simulink model "ESPSIM_Transmission_Multiplex"  (R2025a)
settings: Solver=ode3  StartTime=0.0  StopTime=inf  RelTol=1e-3  EnableMultiTasking=on
libraries: arduinolib x4
settings Model: FPTRunName=Active  SILPILModeSetting=veronly  ExtModeTrigDuration=2  Creator=antho  LastModifiedBy=antho
settings SolverCC: AlgebraicLoopSolver=TrustRegion  AutoInsertRateTranBlk=on
settings DataIOCC: LimitDataPoints=on  SaveFormat=Array
settings OptimizationCC: ReuseModelBlockBuffer=off  ExpressionDepthLimit=2147483647.0  LifeSpan=Inf  MaxStackSize=64
settings DebuggingCC: UnderspecifiedInitializationDetection=Classic  MergeDetectMultiDrivingBlocksExec=none  FcnCallInpInsideContextMsg=warning  UnconnectedInputMsg=warning  UnconnectedOutputMsg=warning  UnconnectedLineMsg=warning  AllowSymbolicDim=off  StateNameClashWarn=warning  SFUnexpectedBacktrackingDiag=warning  SFNoUnconditionalDefaultTransitionDiag=warning  SFExecutionAtInitializationDiag=none  ArithmeticOperatorsInVariantConditions=warning
settings HardwareCC: ProdBitPerPointer=32.0  ProdBitPerSizeT=32.0  ProdBitPerPtrDiffT=32.0  ProdLargestAtomicInteger=Long  ProdLargestAtomicFloat=Double  ProdWordSize=32.0  ProdHWDeviceType=ARM Compatible->ARM Cortex
settings ModelReferenceCC: EnableRefExpFcnMdlSchedulingChecks=on  PropagateSignalLabelsOutOfModel=off
settings SFSimCC: SimUseLocalCustomCode=off  CustomCodeUndefinedFunction=UseInterfaceOnly
settings RTWCC: SystemTargetFile=ert.tlc  HardwareBoard=ESP32-WROOM (Arduino Compatible)  TemplateMakefile=ert_default_tmf  GenerateReport=on  RTWVerbose=off  RTWUseLocalCustomCode=off  Toolchain=ESP32  BuildConfiguration=Faster Runs  LaunchReport=on  GPUComputeCapability=3.5  Description=Embedded Coder
settings CodeAppCC: ForceParamTrailComments=on  OperatorAnnotations=on  StateflowObjectComments=on  MATLABSourceComments=on
settings ERTTargetCC: ExtModeTransport=3.0  ExtModeAutomaticAllocSize=off  ExtModeStaticAllocSize=65536.0  InlinedParameterPlacement=Hierarchical  DynamicArrayContainerType=coder::array  MultiwordLength=2048.0  ERTCustomFileBanners=off  SupportContinuousTime=on  SupportNonInlinedSFcns=on  RemoveResetFunc=off  SupportVariableSizeSignals=on  ModelStepFunctionPrototypeControlCompliant=off
settings ConfigComp: CovMetricSettings=dw  CovSaveCumulativeToWorkspaceVar=on  CovSaveSingleToWorkspaceVar=on  CovExternalEMLEnable=off  CovSFcnEnable=off

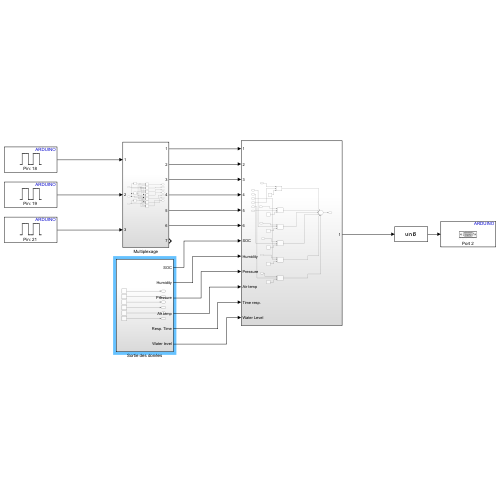
[thumbnail: Simulink's stored preview of the top-level diagram]
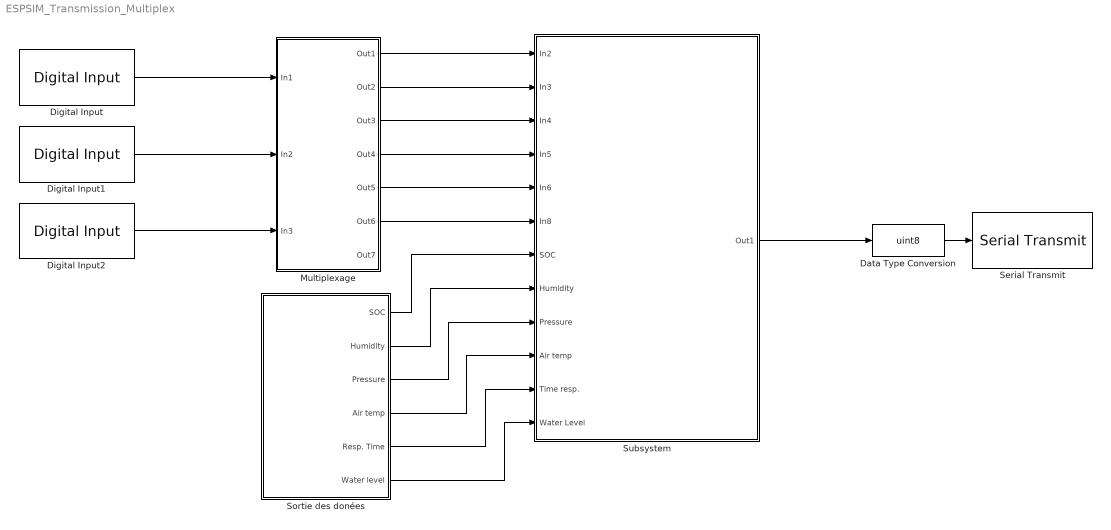
== system ESPSIM_Transmission_Multiplex ==
  Data Type Conversion : DataTypeConversion  OutDataTypeStr=uint8  SaturateOnIntegerOverflow=off  RndMeth=Floor
  Digital Input : arduinolib/Digital Input  pinNumber=18  mode=Default  Direction=input  SampleTime=0.1  blockPlatform=arduino
  Digital Input1 : arduinolib/Digital Input  pinNumber=19  mode=Default  Direction=input  SampleTime=0.1  blockPlatform=arduino
  Digital Input2 : arduinolib/Digital Input  pinNumber=21  mode=Default  Direction=input  SampleTime=0.1  blockPlatform=arduino
  Multiplexage : Subsystem
  Serial Transmit : arduinolib/Serial Transmit  portNumber=2  sendmode=write  sendformat=Binary  floatprecision=1  header=[]  terminator=[]  blockPlatform=ARDUINO
  Sortie des donées : Subsystem
  Subsystem : Subsystem
  wires:
  Data Type Conversion/1 -> Serial Transmit/1
  Digital Input/1 -> Multiplexage/1(In1)
  Digital Input1/1 -> Multiplexage/2(In2)
  Digital Input2/1 -> Multiplexage/3(In3)
  Multiplexage/1(Out1) -> Subsystem/1(In2)
  Multiplexage/2(Out2) -> Subsystem/2(In3)
  Multiplexage/3(Out3) -> Subsystem/3(In4)
  Multiplexage/4(Out4) -> Subsystem/4(In5)
  Multiplexage/5(Out5) -> Subsystem/5(In6)
  Multiplexage/6(Out6) -> Subsystem/6(In8)
  Subsystem/1(Out1) -> Data Type Conversion/1
  Sortie des donées/1(SOC) -> Subsystem/7(SOC)
  Sortie des donées/2(Humidity) -> Subsystem/8(Humidity)
  Sortie des donées/3(Pressure) -> Subsystem/9(Pressure)
  Sortie des donées/4(Air temp) -> Subsystem/10(Air temp)
  Sortie des donées/5(Resp. Time) -> Subsystem/11(Time resp.)
  Sortie des donées/6(Water level) -> Subsystem/12(Water Level)

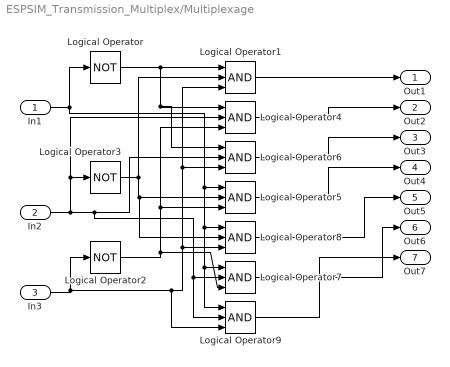
== system ESPSIM_Transmission_Multiplex/Multiplexage ==
  In1 : Inport
  In2 : Inport  Port=2
  In3 : Inport  Port=3
  Logical Operator : Logic  Operator=NOT  AllPortsSameDT=off  OutDataTypeStr=boolean
  Logical Operator{1,4..9} (7 alike) : Logic  Inputs=3  AllPortsSameDT=off  OutDataTypeStr=boolean
  Logical Operator2 : Logic  Operator=NOT  AllPortsSameDT=off  OutDataTypeStr=boolean
  Logical Operator3 : Logic  Operator=NOT  AllPortsSameDT=off  OutDataTypeStr=boolean
  Out1 : Outport
  Out2 : Outport  Port=2
  Out3 : Outport  Port=3
  Out4 : Outport  Port=4
  Out5 : Outport  Port=5
  Out6 : Outport  Port=6
  Out7 : Outport  Port=7
  wires:
  In1/1 -> Logical Operator/1, Logical Operator9/1, Logical Operator7/1, Logical Operator8/1, Logical Operator5/1
  In2/1 -> Logical Operator9/2, Logical Operator7/2, Logical Operator6/2, Logical Operator4/2, Logical Operator3/1
  In3/1 -> Logical Operator9/3, Logical Operator8/3, Logical Operator6/3, Logical Operator1/3, Logical Operator2/1
  Logical Operator/1 -> Logical Operator6/1, Logical Operator4/1, Logical Operator1/1
  Logical Operator3/1 -> Logical Operator8/2, Logical Operator5/2, Logical Operator1/2
  Logical Operator1/1 -> Out1/1
  Logical Operator4/1 -> Out2/1
  Logical Operator6/1 -> Out3/1
  Logical Operator5/1 -> Out4/1
  Logical Operator8/1 -> Out5/1
  Logical Operator7/1 -> Out6/1
  Logical Operator9/1 -> Out7/1
  Logical Operator2/1 -> Logical Operator7/3, Logical Operator5/3, Logical Operator4/3

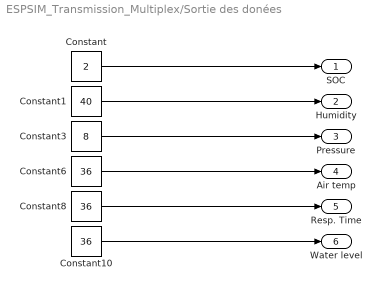
== system ESPSIM_Transmission_Multiplex/Sortie des donées ==
  Constant : Constant  Value=2
  Constant1 : Constant  Value=40
  Constant10 : Constant  Value=36
  Constant3 : Constant  Value=8
  Constant6 : Constant  Value=36
  Constant8 : Constant  Value=36
  SOC : Outport
  Humidity : Outport  Port=2
  Pressure : Outport  Port=3
  Air temp : Outport  Port=4
  Resp. Time : Outport  Port=5
  Water level : Outport  Port=6
  wires:
  Constant10/1 -> Water level/1
  Constant/1 -> SOC/1
  Constant6/1 -> Air temp/1
  Constant8/1 -> Resp. Time/1
  Constant3/1 -> Pressure/1
  Constant1/1 -> Humidity/1

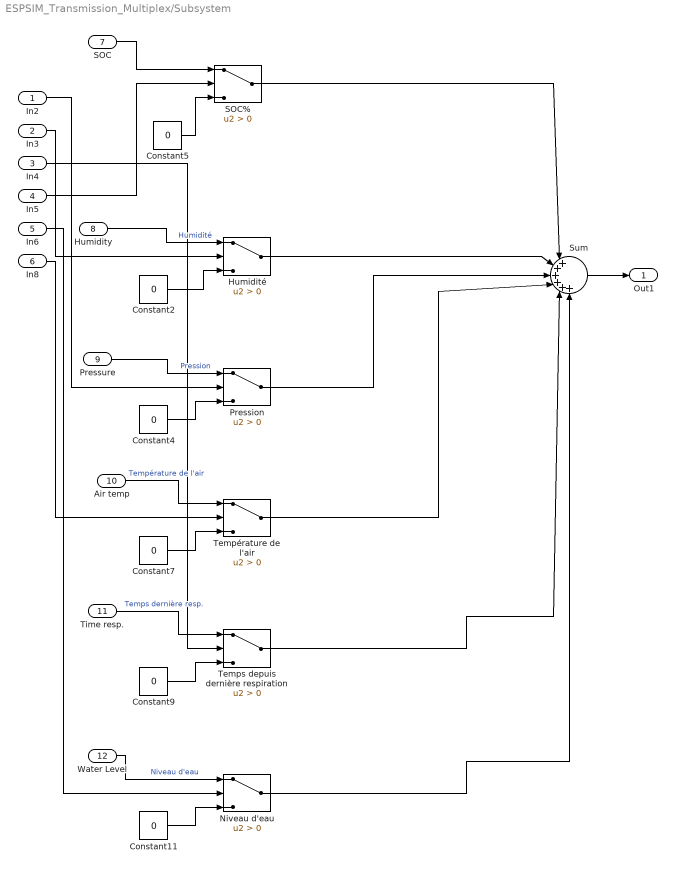
== system ESPSIM_Transmission_Multiplex/Subsystem ==
  In2 : Inport
  In3 : Inport  Port=2
  In4 : Inport  Port=3
  In5 : Inport  Port=4
  In6 : Inport  Port=5
  In8 : Inport  Port=6
  SOC : Inport  Port=7
  Humidity : Inport  Port=8
  Pressure : Inport  Port=9
  Air temp : Inport  Port=10
  Time resp. : Inport  Port=11
  Water Level : Inport  Port=12
  Constant{2,4..5,7,9,11} (6 alike) : Constant  Value=0
  Humidité : Switch  Criteria=u2 > Threshold  SaturateOnIntegerOverflow=off  InputSameDT=off
  Niveau d'eau : Switch  Criteria=u2 > Threshold  SaturateOnIntegerOverflow=off  InputSameDT=off
  Pression : Switch  Criteria=u2 > Threshold  SaturateOnIntegerOverflow=off  InputSameDT=off
  SOC% : Switch  Criteria=u2 > Threshold  SaturateOnIntegerOverflow=off  InputSameDT=off
  Sum : Sum  Inputs=|++++++
  Temps depuis dernière respiration : Switch  Criteria=u2 > Threshold  SaturateOnIntegerOverflow=off  InputSameDT=off
  Température de l'air : Switch  Criteria=u2 > Threshold  SaturateOnIntegerOverflow=off  InputSameDT=off
  Out1 : Outport
  wires:
  SOC%/1 -> Sum/1
  Constant4/1 -> Pression/3
  In6/1 -> Niveau d'eau/2
  Température de l'air/1 -> Sum/4
  Time resp./1 -> Temps depuis dernière respiration/1  "Temps dernière resp."
  Pression/1 -> Sum/3
  Constant11/1 -> Niveau d'eau/3
  Humidité/1 -> Sum/2
  Constant5/1 -> SOC%/3
  Constant2/1 -> Humidité/3
  Air temp/1 -> Température de l'air/1  "Température de l'air"
  Constant7/1 -> Température de l'air/3
  Niveau d'eau/1 -> Sum/6
  Constant9/1 -> Temps depuis dernière respiration/3
  Temps depuis dernière respiration/1 -> Sum/5
  Water Level/1 -> Niveau d'eau/1  "Niveau d'eau"
  Sum/1 -> Out1/1
  In4/1 -> Temps depuis dernière respiration/2
  SOC/1 -> SOC%/1
  In5/1 -> SOC%/2
  In3/1 -> Humidité/2
  Humidity/1 -> Humidité/1  "Humidité"
  Pressure/1 -> Pression/1  "Pression"
  In8/1 -> Température de l'air/2
  In2/1 -> Pression/2
